simulink model "Experimento_Termopar"  (R2021b)
settings: Solver=FixedStepAuto  StartTime=0.0  StopTime=60  RelTol=1e-3  AbsTol=1e-3  EnableMultiTasking=on
libraries: fl_lib x5, nesl_utility x4, raspberrypiCommlib x2, slrealtimeseriallib x1, ee_lib x1
settings Model: Creator=Pc melhor q do euler  LastModifiedBy=Pc melhor q do euler
settings SolverCC: AutoScaleAbsTol=off  AlgebraicLoopSolver=TrustRegion  PositivePriorityOrder=on
settings OptimizationCC: UseDivisionForNetSlopeComputation=on  GainParamInheritBuiltInType=on  UseFloatMulNetSlope=on  PassReuseOutputArgsAs=Individual arguments  ZeroExternalMemoryAtStartup=off  ZeroInternalMemoryAtStartup=off  NoFixptDivByZeroProtection=on  EfficientFloat2IntCast=on  LifeSpan=1  MaxStackSize=64  OptimizeBlockOrder=speed  DifferentSizesBufferReuse=on  EfficientTunableParamExpr=on
settings DebuggingCC: ParameterTunabilityLossMsg=error  SymbolicDimsDataTypeCodeGenerationDiagnostic=none  SFMachineParentedDataDiag=warning
settings HardwareCC: ProdBitPerPointer=32  ProdBitPerSizeT=32  ProdBitPerPtrDiffT=32  ProdLargestAtomicInteger=Long  ProdLargestAtomicFloat=Double  ProdWordSize=32  ProdLongLongMode=on  ProdHWDeviceType=ARM Compatible->ARM Cortex
settings SFSimCC: CustomCodeUndefinedFunction=UseInterfaceOnly
settings RTWCC: Description=Embedded Coder  SystemTargetFile=ert.tlc  HardwareBoard=Raspberry Pi  TLCOptions="-aInlineSetEventsForThisBaseRateFcn=TLC_FALSE -aSuppressMultiTaskScheduler=TLC_FALSE  -aRateBasedStepFcn=0"  TemplateMakefile=ert_default_tmf  Toolchain=GNU GCC Embedded Linux  BuildConfiguration=Faster Runs
settings CodeAppCC: ForceParamTrailComments=on  IgnoreCustomStorageClasses=off  OperatorAnnotations=on  SimulinkDataObjDesc=on  SFDataObjDesc=on  CustomSymbolStrGlobalVar=rt$N$M  CustomSymbolStrType=$N$M  CustomSymbolStrFcn=$N$M$F  CustomSymbolStrMacro=$N$M  InsertBlockDesc=on
settings ERTTargetCC: IncludeMdlTerminateFcn=off  CombineSignalStateStructs=on  SupportComplex=off  SupportContinuousTime=on  SupportVariableSizeSignals=on  ExtModeTransport=2  ExtModeStaticAlloc=on  ExtModeMexFile=ext_xcp  ExtModeIntrfLevel=Level2 - Open  ERTFilePackagingFormat=CompactWithDataFile
settings SimscapeCC: SimscapeLogType=all  SimscapeLogSimulationStatistics=on  SimscapeLogDataHistory=10000

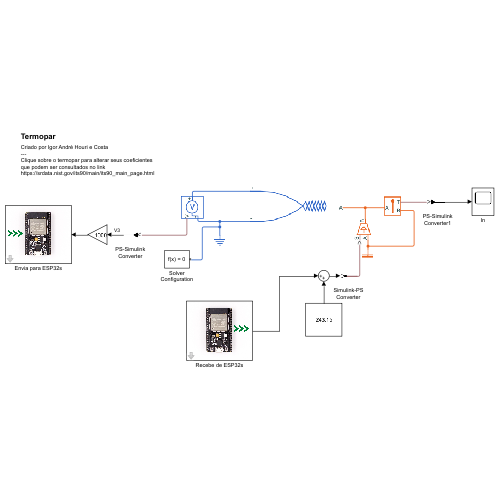
[thumbnail: Simulink's stored preview of the top-level diagram]
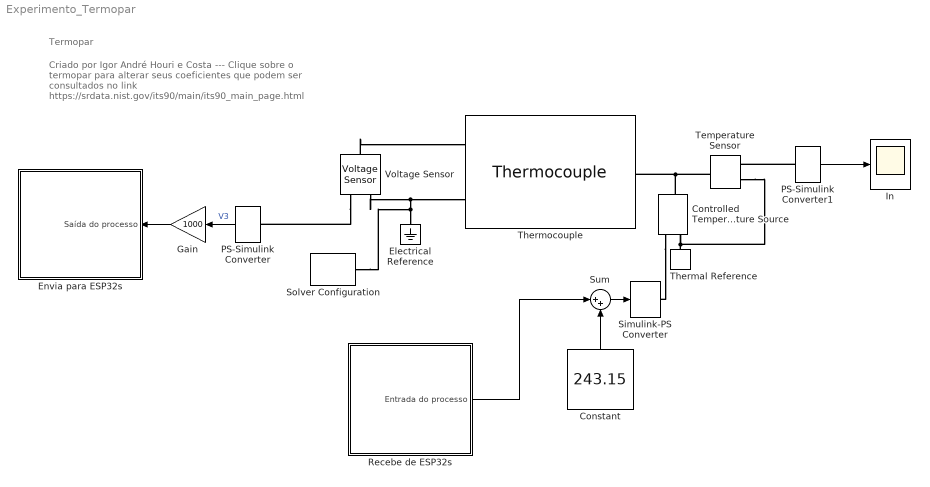
== system Experimento_Termopar ==
  note: Termopar
  note: Criado por Igor André Houri e Costa
      | ---
      | Clique sobre o termopar para alterar seus coeficientes
      | que podem ser consultados no link
      | https://srdata.nist.gov/its90/main/its90_main_page.html
  Constant : Constant  Value=243.15
  Controlled Temperature Source : fl_lib/Thermal/Thermal Sources/Controlled Temperature Source
  Electrical Reference : fl_lib/Electrical/Electrical Elements/Electrical Reference
  Envia para ESP32s : Subsystem  mask(Envio de mensagem Serial - ESP32s){board=Pi 3 Model B, SCIModule_=/dev/ttyS0, Baudrate_=115200, Saida_maxima=0, Saida_minima=-5}
      mask prompts: SCIModule_ "Port:"; Baudrate_ "Baudrate (in bits/s):"; Saida_maxima "Saída máxima do processo"; Saida_minima "Saída mínima do processo"
      mask help: Este bloco recebe em sua entrada um sinal do tipo double, converte-o para a escala necessária e a envia, via mensagem serial, para o ESP32s. --Bloco criado por Igor Costa.
      mask TypeOptions board: Serial Write/board
      mask TypeOptions SCIModule_: Serial Write/SCIModule_
      mask TypeOptions Baudrate_: Serial Write/Baudrate_
      mask TypeOptions Saida_maxima: Função Map (saída)/Saida_maxima
      mask TypeOptions Saida_minima: Função Map (saída)/Saida_minima
      mask Display: image('$imagefile'); % Use "Edit Image" on toolstrip to change.
  Gain : Gain  Gain=1000
  In : Scope
  PS-Simulink Converter : nesl_utility/PS-Simulink Converter  PhysicalDomain=network_engine_domain  SubClassName=ps_output  LeftPortType=input  RightPortType=output  PseudoPeriodic=off  Frequencies=[]  Unit=V  AffineConversion=off
      settings: SourceProductBaseCode=PW,SS
  PS-Simulink Converter1 : nesl_utility/PS-Simulink Converter  PhysicalDomain=network_engine_domain  SubClassName=ps_output  LeftPortType=input  RightPortType=output  PseudoPeriodic=off  Frequencies=[]  Unit=degC  AffineConversion=on
      settings: SourceProductBaseCode=PW,SS
  Recebe de ESP32s : Subsystem  mask(Recepção de mensagem Serial - ESP32s){board=Pi 3 Model B, SCIModule_=/dev/ttyS0, Baudrate_=115200, entrada_maxima=30, entrada_minima=0}
      mask prompts: SCIModule_ "Port:"; Baudrate_ "Baudrate (in bits/s):"; entrada_maxima "Entrada máxima do processo"; entrada_minima "Entrada mínima do processo"
      mask help: Este bloco recebe a mensagem serial enviada pelo ESP32s, decodifica-a e converte para a escala configurada; disponibilizando o resultado em sua saída. --Bloco criado por Igor Costa.
      mask TypeOptions board: Serial Read1/board
      mask TypeOptions SCIModule_: Serial Read1/SCIModule_
      mask TypeOptions Baudrate_: Serial Read1/Baudrate_
      mask TypeOptions entrada_maxima: Função Map (entrada)/entrada_maxima
      mask TypeOptions entrada_minima: Função Map (entrada)/entrada_minima
      mask Display: image('I:\PFC_Igor\plot figuras\figuras\Recebe de ESP32s.png'); % Use "Edit Image" on toolstrip to change.
  Simulink-PS Converter : nesl_utility/Simulink-PS Converter  PhysicalDomain=network_engine_domain  SubClassName=ps_input  LeftPortType=input  RightPortType=output  PseudoPeriodic=off  Frequencies=[]  NoiseDistribution=none  NoiseParameters=[]  Unit=K  AffineConversion=off  FilteringAndDerivatives=filter  SimscapeFilterOrder=1  InputFilterTimeConstant=0.001  UdotUserProvided=0
      settings: SourceProductBaseCode=PW,SS
  Solver Configuration : nesl_utility/Solver Configuration  PhysicalDomain=network_engine_domain  SubClassName=solver  LeftPortType=input  RightPortType=generic  Tones=[]  Harmonics=[]  SimulateNoise=off  Profile=off  UseLocalSampling=off  EnableSwitchedLinearOptims=on  FrequencyDomain=off  UseCCode=off  RelTol=0.001  AbsTol=1e-06  MinStep=1e-09  ToWorkspace=off  RevertToSquareIcSolve=off  NumHomotopyIterations=100  PhasorMode=off  PhasorModeNumHarmonics=1  DoDC=off  ResidualTolerance=1e-09  UseLocalSolver=off  LocalSolverChoice=NE_BACKWARD_EULER_ADVANCER  LocalSolverSampleTime=0.001  DoFixedCost=off  MaxNonlinIter=3  MaxModeIter=2  ComputeImpulses=off  ImpulseIterations=2  LinearAlgebra=auto  EquationFormulation=NE_TIME_EF  DelaysMemoryBudget=1024  AutomaticFiltering=on  FilteringTimeConstant=0.001  PartitionStorageMethod=AS_NEEDED  PartitionMemoryBudget=1024  PartitionMethod=ROBUST
      settings: SourceProductBaseCode=PW,SS
  Sum : Sum  Inputs=|++
  Temperature Sensor : fl_lib/Thermal/Thermal Sensors/Temperature Sensor
  Thermal Reference : fl_lib/Thermal/Thermal Elements/Thermal Reference
  Thermocouple : ee_lib/Sensors & Transducers/Thermocouple  thermocouple_type=1  Cvec=[0.000000000000,0.394501280250e-1,0.236223735980e-4,-0.328589067840e-6,-0.499048287770e-8,-0.67509059173e-10,-0.574103274280e-12,-0.310888728940e-14,-0.104516093650e-16,-0.198892668780e-19,-0.163226974860e-22]  Avec=[0.118597600000, -0.118343200000e-3, 0.126968600000e3]  T0=0 degC  tc=1 hr  K_d=1e-3 W/K  init_temp=20 degC
      settings: SourceProductBaseCode=PS  InternalSimscapePortConfiguration="{\"Bottom\":[],\"Left\":[{\"id\":\"p\",\"label\":\"+\",\"type\":\"foundation.electrical.electrical\"},{\"id\":\"n\",\"label\":\"-\",\"type\":\"foundation.electrical.electrical\"}],\"Right\":[{\"id\":\"A\",\"label\":\"A\",\"type\":\"foundation.thermal.thermal\"}],\"Top\":[]}"
  Voltage Sensor : fl_lib/Electrical/Electrical Sensors/Voltage Sensor
  wires:
  PS-Simulink Converter/1 -> Gain/1  "V3"
  Gain/1 -> Envia para ESP32s/1(Saída do processo)
  PS-Simulink Converter1/1 -> In/1
  Sum/1 -> Simulink-PS Converter/1
  Constant/1 -> Sum/2
  Recebe de ESP32s/1(Entrada do processo) -> Sum/1
  connections:
  Voltage Sensor/LConn1 -- Thermocouple/LConn1
  Voltage Sensor/RConn2 -- Thermocouple/LConn2 -- Solver Configuration/RConn1 -- Electrical Reference/LConn1
  Voltage Sensor/RConn1 -- PS-Simulink Converter/LConn1
  Thermal Reference/LConn1 -- Temperature Sensor/RConn1 -- Controlled Temperature Source/RConn2
  Controlled Temperature Source/LConn1 -- Thermocouple/RConn1 -- Temperature Sensor/LConn1
  Controlled Temperature Source/RConn1 -- Simulink-PS Converter/RConn1
  PS-Simulink Converter1/LConn1 -- Temperature Sensor/RConn2

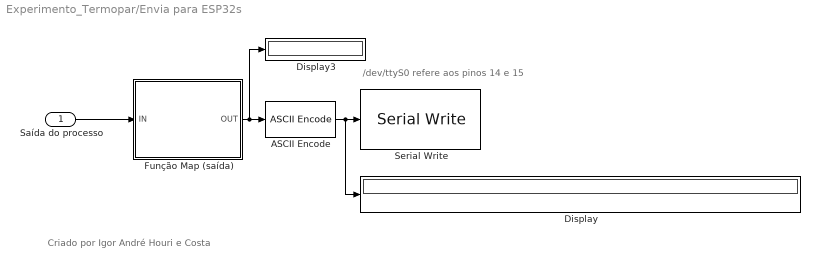
== system Experimento_Termopar/Envia para ESP32s ==
  note: /dev/ttyS0 refere aos pinos 14 e 15
  note: Criado por Igor André Houri e Costa
  Saída do processo : Inport
  ASCII Encode : slrealtimeseriallib/ASCII Encode  format=%d\r  nvars=1  maxlength=32  vartypes={ 'double' }
      settings: SourceProductBaseCode=XP
  Display : Display
  Display3 : Display
  Função Map (saída) : Subsystem  mask(Função Map - entrada){Saida_maxima=Saida_maxima, Saida_minima=Saida_minima}
      mask prompts: Saida_maxima "Saída máxima do processo"; Saida_minima "Saída mínima do processo"
      mask help: Este bloco mapeia um número de uma escala (range) para a escala necessária para envio da saída do processo ao ESP32s (0 a 4095). A função implementada é (x - x_min) * (4095 - 0) / (x_max - x_min) + 0, sendo "x" o valor do número a ser mapeado, "x_min" o menor valor possível para x e "x_max" o maior valor possível para x. --Bloco criado por Igor Costa.
      mask Help: sdsd
      mask TypeOptions Saida_maxima: Saida_maxima/Value
      mask TypeOptions Saida_minima: Saida_minima/Value
  Serial Write : raspberrypiCommlib/Serial Write  board=Pi 3 Model B  SCIModule_=/dev/ttyS0  Baudrate_=115200  Parity=None  StopBits_=1  HardwareFlowControl=None  ByteOrder=LittleEndian  OutputStatus=off  blockPlatform=RaspberryPi
      settings: SourceProductBaseCode=RASPPI
  wires:
  Função Map (saída)/1(OUT) -> Display3/1, ASCII Encode/1
  ASCII Encode/1 -> Display/1, Serial Write/1
  Saída do processo/1 -> Função Map (saída)/1(IN)

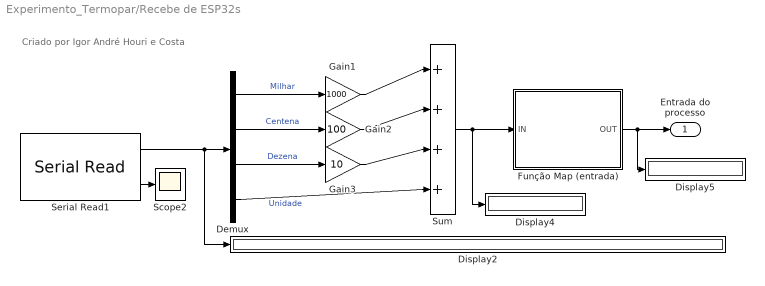
== system Experimento_Termopar/Recebe de ESP32s ==
  note: Criado por Igor André Houri e Costa
  Demux : Demux
  Display2 : Display
  Display4 : Display
  Display5 : Display
  Função Map (entrada) : Subsystem  mask(Função Map - entrada){entrada_maxima=entrada_maxima, entrada_minima=entrada_minima}
      mask prompts: entrada_maxima "Entrada máxima do processo"; entrada_minima "Entrada mínima do processo"
      mask help: Este bloco mapeia um número de uma escala (range) da escala necessária para decodificação da entrada do processo recebida ESP32s (0 a 4095), passando-o para a escala dos valores do processo. A função implementada é (x - 0) * (x_max - x_min) / (4095 - 0), sendo "x" o valor do número a ser mapeado, "x_min" o menor valor possível para x e "x_max" o maior valor possível para x. --Bloco criado por Igor Costa.
      mask TypeOptions entrada_maxima: Entrada_maxima/Value
      mask TypeOptions entrada_minima: Entrada_minima/Value
  Gain1 : Gain  Gain=1000
  Gain2 : Gain  Gain=100
  Gain3 : Gain  Gain=10
  Scope2 : Scope
  Serial Read1 : raspberrypiCommlib/Serial Read  board=Pi 3 Model B  SCIModule_=/dev/ttyS0  Baudrate_=115200  Parity=None  StopBits_=1  HardwareFlowControl=None  ByteOrder=LittleEndian  DataLength=4  DataType=uint8  OutputStatus=on  SampleTime=0.1  blockPlatform=RaspberryPi
      settings: SourceProductBaseCode=RASPPI
  Sum : Sum  Inputs=|++++
  Entrada do processo : Outport
  wires:
  Demux/3 -> Gain3/1  "Dezena"
  Demux/4 -> Sum/4  "Unidade"
  Demux/2 -> Gain2/1  "Centena"
  Serial Read1/2 -> Scope2/1
  Demux/1 -> Gain1/1  "Milhar"
  Sum/1 -> Display4/1, Função Map (entrada)/1(IN)
  Gain1/1 -> Sum/1
  Gain2/1 -> Sum/2
  Serial Read1/1 -> Display2/1, Demux/1
  Gain3/1 -> Sum/3
  Função Map (entrada)/1(OUT) -> Display5/1, Entrada do processo/1

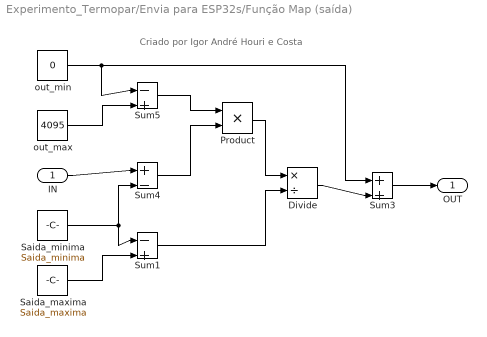
== system Experimento_Termopar/Envia para ESP32s/Função Map (saída) ==
  note: Criado por Igor André Houri e Costa
  IN : Inport
  Divide : Product  Inputs=*/
  Product : Product
  Saida_maxima : Constant  Value=Saida_maxima
  Saida_minima : Constant  Value=Saida_minima
  Sum1 : Sum  Inputs=|-+
  Sum3 : Sum  Inputs=++|
  Sum4 : Sum  Inputs=|+-
  Sum5 : Sum  Inputs=|-+
  out_max : Constant  Value=4095
  out_min : Constant  Value=0
  OUT : Outport
  wires:
  Sum5/1 -> Product/1
  out_max/1 -> Sum5/2
  Sum1/1 -> Divide/2
  Saida_minima/1 -> Sum4/2, Sum1/1
  IN/1 -> Sum4/1
  out_min/1 -> Sum3/1, Sum5/1
  Divide/1 -> Sum3/2
  Sum4/1 -> Product/2
  Product/1 -> Divide/1
  Sum3/1 -> OUT/1
  Saida_maxima/1 -> Sum1/2

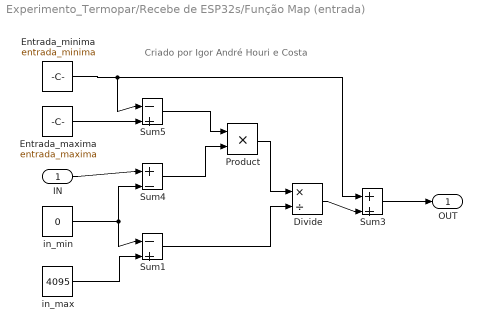
== system Experimento_Termopar/Recebe de ESP32s/Função Map (entrada) ==
  note: Criado por Igor André Houri e Costa
  IN : Inport
  Divide : Product  Inputs=*/
  Entrada_maxima : Constant  Value=entrada_maxima
  Entrada_minima : Constant  Value=entrada_minima
  Product : Product
  Sum1 : Sum  Inputs=|-+
  Sum3 : Sum  Inputs=++|
  Sum4 : Sum  Inputs=|+-
  Sum5 : Sum  Inputs=|-+
  in_max : Constant  Value=4095
  in_min : Constant  Value=0
  OUT : Outport
  wires:
  Sum5/1 -> Product/1
  Sum1/1 -> Divide/2
  IN/1 -> Sum4/1
  Entrada_minima/1 -> Sum3/1, Sum5/1
  Divide/1 -> Sum3/2
  Sum4/1 -> Product/2
  Product/1 -> Divide/1
  Sum3/1 -> OUT/1
  in_max/1 -> Sum1/2
  in_min/1 -> Sum1/1, Sum4/2
  Entrada_maxima/1 -> Sum5/2
